simulink model "ConstrainedSphereModel"  (R2017b)
settings: Solver=VariableStepAuto  StartTime=0.0  StopTime=12  RelTol=1e-3
undefined symbols (not defined in the file): b_contact, C_F_alpha, C_F_kappa, g, k_contact, radiusRW, sigbuilder_block, theta_0, X, xPla, Y, yPla, Z
libraries: nesl_utility x15, sm_lib x7, vrlib x7, Parts_Lib x1, simulink x1
settings Model: Creator=r_ahmed_afzal  LastModifiedBy=r_ahmed_afzal

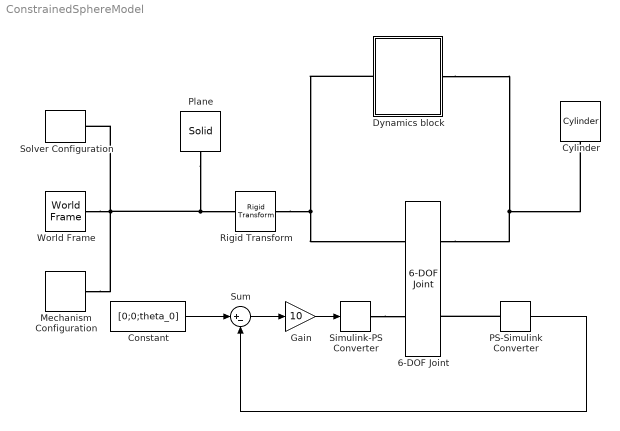
== system ConstrainedSphereModel ==
  6-DOF Joint : sm_lib/Joints/6-DOF Joint  SenseConstraintForce=off  SenseConstraintForceX=off  SenseConstraintForceY=off  SenseConstraintForceZ=off  SenseConstraintTorque=off  SenseConstraintTorqueX=off  SenseConstraintTorqueY=off  SenseConstraintTorqueZ=off  SenseTotalForce=off  SenseTotalForceX=off  SenseTotalForceY=off  SenseTotalForceZ=off  SenseTotalTorque=off  SenseTotalTorqueX=off  SenseTotalTorqueY=off  SenseTotalTorqueZ=off  CompositeWrenchDir=FollowerOnBase  CompositeWrenchFrame=BaseFrame  PxEquilibriumPosition=0  PxEquilibriumPositionUnits=m  PxSpringStiffness=0  PxSpringStiffnessUnits=N/m  PxDampingCoefficient=0  PxDampingCoefficientUnits=N/(m/s)  PxTorqueActuationMode=NoTorque  PxMotionActuationMode=ComputedMotion  PxSensePosition=off  PxSenseVelocity=off  PxSenseAcceleration=off  PxSenseTorqueForce=off  PxPositionTargetSpecify=on  PxPositionTargetPriority=High  PxPositionTargetValue=radiusRW  PxPositionTargetValueUnits=m  PxVelocityTargetSpecify=off  PxVelocityTargetPriority=High  PxVelocityTargetValue=0  PxVelocityTargetValueUnits=m/s  PyEquilibriumPosition=0  PyEquilibriumPositionUnits=m  PySpringStiffness=0  PySpringStiffnessUnits=N/m  PyDampingCoefficient=0  PyDampingCoefficientUnits=N/(m/s)  PyTorqueActuationMode=NoTorque  PyMotionActuationMode=ComputedMotion  PySensePosition=off  PySenseVelocity=off  PySenseAcceleration=off  PySenseTorqueForce=off  PyPositionTargetSpecify=on  PyPositionTargetPriority=High  PyPositionTargetValue=-xPla/2 + 0.1  PyPositionTargetValueUnits=m  PyVelocityTargetSpecify=off  PyVelocityTargetPriority=High  PyVelocityTargetValue=0  PyVelocityTargetValueUnits=m/s  PzEquilibriumPosition=0  PzEquilibriumPositionUnits=m  PzSpringStiffness=0  PzSpringStiffnessUnits=N/m  PzDampingCoefficient=0  PzDampingCoefficientUnits=N/(m/s)  PzTorqueActuationMode=NoTorque  PzMotionActuationMode=ComputedMotion  PzSensePosition=off  PzSenseVelocity=off  PzSenseAcceleration=off  PzSenseTorqueForce=off  PzPositionTargetSpecify=off  PzPositionTargetPriority=High  PzPositionTargetValue=0  PzPositionTargetValueUnits=m  PzVelocityTargetSpecify=off  PzVelocityTargetPriority=High  PzVelocityTargetValue=0  PzVelocityTargetValueUnits=m/s  SphDefPosRotationMethod=None  SphDefPosRotationAngleUnits=deg  SphDefPosRotationStandardAxis=+Z  SphDefPosRotationAngle=0.0  SphDefPosRotationArbitraryAxis=[0 0 1]  SphDefPosFollAlignAxisA=+X  SphDefPosBaseAlignAxisA=+Y  SphDefPosFollAlignAxisB=+Y  SphDefPosBaseAlignAxisB=+Z  SphDefPosRotationSequenceAxes=FollowerAxes  SphDefPosRotationSequence=XYX  SphDefPosRotationSequenceAngles=[0 0 0]  SphDefPosRotationSequenceAnglesUnits=deg  SphDefPosRotationMatrix=[1 0 0; 0 1 0; 0 0 1]  SphEqPosRotationMethod=None  SphEqPosRotationAngleUnits=deg  SphEqPosRotationStandardAxis=+Z  SphEqPosRotationAngle=0.0  SphEqPosRotationArbitraryAxis=[0 0 1]  SphEqPosFollAlignAxisA=+X  SphEqPosBaseAlignAxisA=+Y  SphEqPosFollAlignAxisB=+Y  SphEqPosBaseAlignAxisB=+Z  SphEqPosRotationSequenceAxes=FollowerAxes  SphEqPosRotationSequence=XYX  SphEqPosRotationSequenceAngles=[0 0 0]  SphEqPosRotationSequenceAnglesUnits=deg  SphEqPosRotationMatrix=[1 0 0; 0 1 0; 0 0 1]  SphSpringStiffness=0  SphSpringStiffnessUnits=N*m/deg  SphDampingCoefficient=0  SphDampingCoefficientUnits=N*m/(deg/s)  SphActuateTorqueX=off  SphActuateTorqueY=off  SphActuateTorqueZ=off  SphActuateTorque=on  SphTorqueActuationMode=InputTorque  SphMotionActuationMode=ComputedMotion  SphActuationFrame=FollowerFrame  SphSensePosition=off  SphSenseVelocityX=off  SphSenseVelocityY=off  SphSenseVelocityZ=off  SphSenseVelocity=on  SphSenseAccelerationX=off  SphSenseAccelerationY=off  SphSenseAccelerationZ=off  SphSenseAcceleration=off  SphSenseTorqueX=off  SphSenseTorqueY=off  SphSenseTorqueZ=off  SphSenseTorqueForce=off  SphSensingFrame=FollowerFrame  SphPositionTargetRotationMethod=StandardAxis  SphPositionTargetRotationAngleUnits=deg  SphPositionTargetRotationStandardAxis=+Y  SphPositionTargetRotationAngle=5  SphPositionTargetRotationArbitraryAxis=[0 0 1]  SphPositionTargetFollAlignAxisA=+X  SphPositionTargetBaseAlignAxisA=+Y  SphPositionTargetFollAlignAxisB=+Y  SphPositionTargetBaseAlignAxisB=+Z  SphPositionTargetRotationSequenceAxes=FollowerAxes  SphPositionTargetRotationSequence=XYX  SphPositionTargetRotationSequenceAngles=[0 0 0]  SphPositionTargetRotationSequenceAnglesUnits=deg  SphPositionTargetRotationMatrix=[1 0 0; 0 1 0; 0 0 1]  SphPositionTargetSpecify=on  SphPositionTargetPriority=High  SphVelocityTargetValue=[0 0 0]  SphVelocityTargetValueUnits=deg/s  SphVelocityTargetSpecify=off  SphVelocityTargetPriority=High  SphVelocityTargetInFollowerFrame=on
  Constant : Constant  Value=[0;0;theta_0]
  Cylinder : Parts_Lib/Cylinder  Tag=CustomStyle  cyl_radius=radiusRW  cyl_length=lengthRW  cyl_density=rhoRW  cyl_color=blue  cyl_opacity=1  cyl_color_custom="[0.7920    0.9900    0.9900]"  mark_radius=[0.75 0.5]  mark_len_factor=1.01  mark_angle=60  mark_color=purple  mark_opacity=1
  Dynamics block : Subsystem
  Gain : Gain  Gain=10
  Mechanism Configuration : sm_lib/Utilities/Mechanism Configuration  UniformGravity=Constant  GravityVector=[0 0 -g]  GravityUnits=m/s^2  LinearizationDelta=0.001
  PS-Simulink Converter : nesl_utility/PS-Simulink Converter  PhysicalDomain=network_engine_domain  SubClassName=ps_output  LeftPortType=input  RightPortType=output  PseudoPeriodic=off  Frequencies=[]  Unit=1  AffineConversion=off
  Plane : sm_lib/Body Elements/Solid  InertiaType=CalculateFromGeometry  Mass=1  MassUnits=kg  CenterOfMass=[0 0 0]  CenterOfMassUnits=m  MomentsOfInertia=[1 1 1]  MomentsOfInertiaUnits=kg*m^2  ProductsOfInertia=[1 1 1]  ProductsOfInertiaUnits=kg*m^2  DensityBased=on  Density=1000  DensityUnits=kg/m^3  DoExposeReferenceFrame=on  SerializedFrames=<Frames/>  GraphicType=FromGeometry  MarkerShape=Sphere  MarkerSize=10  GraphicVisPropType=SimpleVisualProperties  GraphicDiffuseColor=[0.5 0.5 0.5]  GraphicSpecularColor=[0.5 0.5 0.5 1.0]  GraphicAmbientColor=[0.15 0.15 0.15 1.0]  GraphicEmissiveColor=[0.0 0.0 0.0 1.0]  GraphicShininess=75  GraphicOpacity=0.5  GeometryShape=Brick  RectangleSize=[1 1]  RectangleSizeUnits=m  BrickDimensions=[xPla yPla 0.01]  BrickDimensionUnits=m  CylinderRadius=1  CylinderRadiusUnits=m  CylinderLength=1  CylinderLengthUnits=m  SphereRadius=1  SphereRadiusUnits=m  EllipsoidRadii=[1 1 1]  EllipsoidRadiiUnits=m  ExtrusionCrossSection=[1 1; -1 1; -1 -1; 1 -1]  ExtrusionCrossSectionUnits=m  ExtrusionLength=1  ExtrusionLengthUnits=m  PolygonNumSides=3  PolygonOuterRadius=1  PolygonOuterRadiusUnits=m  ExtGeomFileType=STEP  ExtGeomFileUnits=m  RevolutionCrossSection=[1 1; 1 -1; 2 -1; 2 1]  RevolutionCrossSectionUnits=m  RevolutionExtent=Full  RevolutionAngle=180  RevolutionAngleUnits=deg
  Rigid Transform : sm_lib/Frames and Transforms/Rigid Transform  TranslationMethod=None  TranslationStandardOffset=0  TranslationLengthUnit=m  TranslationStandardAxis=+Z  TranslationCartesianOffset=[0 0 0]  TranslationROffset=0  TranslationROffsetUnits=m  TranslationZOffset=0  TranslationZOffsetUnits=m  TranslationThetaOffset=0  TranslationThetaOffsetUnits=deg  RotationMethod=AlignedAxes  RotationAngleUnits=deg  RotationStandardAxis=+Z  RotationAngle=0.0  RotationArbitraryAxis=[0 0 1]  FollAlignAxisA=+Z  BaseAlignAxisA=+Y  FollAlignAxisB=+Y  BaseAlignAxisB=+X  RotationSequenceAxes=FollowerAxes  RotationSequence=XYX  RotationSequenceAngles=[0 0 0]  RotationSequenceAnglesUnits=deg  RotationMatrix=[1 0 0; 0 1 0; 0 0 1]
  Simulink-PS Converter : nesl_utility/Simulink-PS Converter  PhysicalDomain=network_engine_domain  SubClassName=ps_input  LeftPortType=input  RightPortType=output  PseudoPeriodic=off  Frequencies=[]  NoiseDistribution=none  NoiseParameters=[]  Unit=1  AffineConversion=off  FilteringAndDerivatives=filter  SimscapeFilterOrder=2  InputFilterTimeConstant=0.001  UdotUserProvided=0
  Solver Configuration : nesl_utility/Solver Configuration  PhysicalDomain=network_engine_domain  SubClassName=solver  LeftPortType=input  RightPortType=generic  Accelerate=off  Tones=[]  Harmonics=[]  SimulateNoise=off  Profile=off  UseLocalSampling=off  EnableSwitchedLinearOptims=on  FrequencyDomain=off  UseCCode=off  RelTol=0.001  AbsTol=1e-06  MinStep=1e-09  ToWorkspace=off  RevertToSquareIcSolve=off  NumHomotopyIterations=100  PhasorMode=off  PhasorModeNumHarmonics=1  DoDC=off  ResidualTolerance=1e-09  UseLocalSolver=off  LocalSolverChoice=NE_BACKWARD_EULER_ADVANCER  LocalSolverSampleTime=0.001  DoFixedCost=off  MaxNonlinIter=3  MaxModeIter=2  LinearAlgebra=Sparse  DelaysMemoryBudget=1024  AutomaticFiltering=on  FilteringTimeConstant=0.001
  Sum : Sum  Inputs=|+-
  World Frame : sm_lib/Frames and Transforms/World Frame
  wires:
  Constant/1 -> Sum/1
  PS-Simulink Converter/1 -> Sum/2
  Sum/1 -> Gain/1
  Gain/1 -> Simulink-PS Converter/1
  connections:
  Mechanism Configuration/RConn1 -- World Frame/RConn1 -- Rigid Transform/LConn1 -- Plane/RConn1 -- Solver Configuration/RConn1
  Simulink-PS Converter/RConn1 -- 6-DOF Joint/LConn2
  Rigid Transform/RConn1 -- Dynamics block/LConn1 -- 6-DOF Joint/LConn1
  Cylinder/LConn1 -- Dynamics block/RConn1 -- 6-DOF Joint/RConn1
  PS-Simulink Converter/LConn1 -- 6-DOF Joint/RConn2

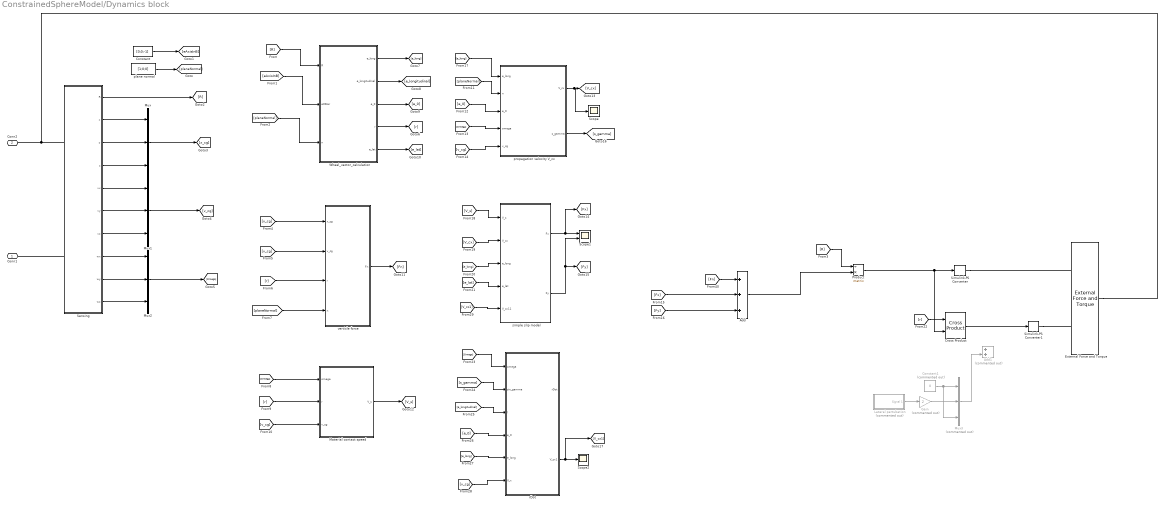
== system ConstrainedSphereModel/Dynamics block ==
  Add : Sum  Inputs=3
  Add1 : Sum  Commented=on
  Constant : Constant  Value=[0;0;-1]
  Constant1 : Constant  Commented=on  Value=0
  Cross Product : vrlib/Utilities/Cross Product
      settings: SourceProductBaseCode=VR
  External Force and Torque : sm_lib/Forces and Torques/External Force and Torque  ForceResolutionFrame=AttachedFrame  EnableForceX=off  EnableForceY=off  EnableForceZ=off  EnableForce=on  TorqueResolutionFrame=AttachedFrame  EnableTorqueX=off  EnableTorqueY=off  EnableTorqueZ=off  EnableTorque=on
  Gain : Gain  Commented=on  Gain=2
  Lateral pertubation : Subsystem  Tag=STV Subsys  Commented=on  LoadFcn=sigbuilder_block('load');  StartFcn=sigbuilder_block('start');  StopFcn=sigbuilder_block('stop');  ClipboardFcn=sigbuilder_block('clipboard');  mask(Sigbuilder block){tuvar=[0:10]}
      mask help: Simulink:masks:SigbuilderBlock_MD
      mask init:
      | if ~strcmp(get_param(bdroot(gcbh),'SimulationStatus'),'stopped') tuvar = sigbuilder_block('maskInit'); end
      settings: CopyFcn=sigbuilder_block('copy');  DeleteFcn=sigbuilder_block('delete');  ModelCloseFcn=sigbuilder_block('modelClose');  PreSaveFcn=sigbuilder_block('preSave');  PauseFcn=sigbuilder_block('pause');  ContinueFcn=sigbuilder_block('continue');  NameChangeFcn=sigbuilder_block('namechange');  OpenFcn=sigbuilder_block('open',[437.6 199.2 550.4 400 ]);  CloseFcn=sigbuilder_block('close');
      mask Display: plot(0, 0, 100, 100,[2, 2, 32, 32, 2], [68, 8, 8, 68, 68],[32, 2], [38, 38], [32, 19, 2],[53, 60, 44], [32, 17, 17, 2],[16, 16, 31, 31]);txt = getActiveGroup(gcbh);text(2, 100, txt,'verticalAlignment', 'top');
  Material contact speed : Subsystem
  Mux : Mux  Inputs=3
  Mux1 : Mux  Inputs=3
  Mux2 : Mux  Inputs=3
  Mux3 : Mux  Commented=on  Inputs=3
  Product : Product  Inputs=/*  Multiplication=Matrix(*)
  Scope : Scope
  Scope1 : Scope  NumInputPorts=2
  Scope2 : Scope
  Sensing : Subsystem
  Simulink-PS Converter : nesl_utility/Simulink-PS Converter  PhysicalDomain=network_engine_domain  SubClassName=ps_input  LeftPortType=input  RightPortType=output  PseudoPeriodic=off  Frequencies=[]  NoiseDistribution=none  NoiseParameters=[]  Unit=1  AffineConversion=off  FilteringAndDerivatives=provide  SimscapeFilterOrder=1  InputFilterTimeConstant=0.001  UdotUserProvided=0
  Simulink-PS Converter1 : nesl_utility/Simulink-PS Converter  PhysicalDomain=network_engine_domain  SubClassName=ps_input  LeftPortType=input  RightPortType=output  PseudoPeriodic=off  Frequencies=[]  NoiseDistribution=none  NoiseParameters=[]  Unit=1  AffineConversion=off  FilteringAndDerivatives=provide  SimscapeFilterOrder=1  InputFilterTimeConstant=0.001  UdotUserProvided=0
  Wheel_vector_calculation : Subsystem
  plane normal : Constant  Value=[1;0;0]
  propagation velocity V_cx : Subsystem
  rDot : Subsystem
  simple slip model : Subsystem
  verticle force : Subsystem
  Conn1 : PMIOPort  Port=1  Side=Left
  Conn2 : PMIOPort  Port=2  Side=Right
  wires:
  plane normal/1 -> [planeNormal]
  Constant/1 -> [eAxisInB]
  Sensing/1(R) -> [R]
  Sensing/2(x) -> Mux/1
  Sensing/3(y) -> Mux/2
  Sensing/4(z) -> Mux/3
  Mux/1 -> [x_cg]
  Sensing/6(vy) -> Mux1/2
  Sensing/5(vx) -> Mux1/1
  Sensing/7(vz) -> Mux1/3
  Mux1/1 -> [v_cg]
  Sensing/9(wy) -> Mux2/2
  Sensing/8(wx) -> Mux2/1
  Sensing/10(wz) -> Mux2/3
  Mux2/1 -> [Omega]
  [R] -> Product/1
  Product/1 -> Cross Product/2, Simulink-PS Converter/1
  [R] -> Wheel_vector_calculation/1(R)
  [eAxisInB] -> Wheel_vector_calculation/2(e0Star)
  [planeNormal] -> Wheel_vector_calculation/3(n)
  [x_cg] -> verticle force/1(x_cg)
  [v_cg] -> verticle force/2(v_cg)
  Wheel_vector_calculation/4(r) -> [r]
  Wheel_vector_calculation/1(e_long) -> [e_long]
  Wheel_vector_calculation/2(e_longitudinal) -> [e_longitudinal]
  Wheel_vector_calculation/3(e_0) -> [e_0]
  Wheel_vector_calculation/5(e_lat) -> [e_lat]
  [r] -> verticle force/3(r)
  [planeNormal] -> verticle force/4(n)
  verticle force/1(Fn) -> [Fn]
  [Omega] -> Material contact speed/1(omega)
  [r] -> Material contact speed/2(r)
  [v_cg] -> Material contact speed/3(v_cg)
  Material contact speed/1(V_s) -> [V_s]
  [Fn] -> Add/1
  [Fx] -> Add/2
  [Fy] -> Add/3
  [planeNormal] -> propagation velocity V_cx/2(n)
  [e_0] -> propagation velocity V_cx/3(e_0)
  [Omega] -> propagation velocity V_cx/4(omega)
  [v_cg] -> propagation velocity V_cx/5(v_cg)
  [e_long] -> propagation velocity V_cx/1(e_long)
  propagation velocity V_cx/1(V_cx) -> Scope/1, [V_cx]
  [V_s] -> simple slip model/1(V_s)
  [V_cx] -> simple slip model/2(V_cx)
  [e_long] -> simple slip model/3(e_long)
  [e_lat] -> simple slip model/4(e_lat)
  simple slip model/2(Fy) -> [Fy], Scope1/2
  Lateral pertubation/1(Signal 1) -> Gain/1
  Mux3/1 -> Add1/2
  Add/1 -> Product/2
  Gain/1 -> Mux3/2
  Constant1/1 -> Mux3/3, Mux3/1
  [r] -> Cross Product/1
  [Omega] -> rDot/1(omega)
  propagation velocity V_cx/2(s_gamma) -> [s_gamma]
  [s_gamma] -> rDot/2(sin_gamma)
  [e_longitudinal] -> rDot/3(l)
  [e_0] -> rDot/4(e_0)
  [e_long] -> rDot/5(e_long)
  [v_cg] -> rDot/6(V_x)
  rDot/2(V_cx1) -> [V_cx1], Scope2/1
  [V_cx1] -> simple slip model/5(V_cx11)
  simple slip model/1(Fx) -> [Fx], Scope1/1
  Cross Product/1 -> Simulink-PS Converter1/1
  connections:
  Sensing/LConn1 -- External Force and Torque/RConn1 -- Conn2/RConn1
  Sensing/LConn2 -- Conn1/RConn1
  Simulink-PS Converter/RConn1 -- External Force and Torque/LConn1
  Simulink-PS Converter1/RConn1 -- External Force and Torque/LConn2

== system ConstrainedSphereModel/Dynamics block/Lateral pertubation ==
  Demux : Demux  Tag=STV Demux  Outputs=1
  FromWs : FromWorkspace  Tag=STV FromWs  VariableName=tuvar  SampleTime=0
      SigBuilderData=|
      | common.afterFinalStr = 'Extrapolate'
      | common.sampleTime = 0
      | dataSet.timeRange = [0 10]
      | dataSet.name = 'Group 1'
      | sbobj.Groups.Name = 'Group 1'
      | sbobj.Groups.Signals.Name = 'Signal 1'
      | sbobj.Groups.Signals.XData = [0 1 1 1.5 1.5 10]
      | sbobj.Groups.Signals.YData = [0 0 1 1 0 0]
  Signal 1 : Outport  Tag=STV Outport
  wires:
  Demux/1 -> Signal 1/1
  FromWs/1 -> Demux/1

== system ConstrainedSphereModel/Dynamics block/Material contact speed ==
  omega : Inport
  r : Inport  Port=2
  v_cg : Inport  Port=3
  Cross Product : vrlib/Utilities/Cross Product
      settings: SourceProductBaseCode=VR
  Sum : Sum  Inputs=|++
  V_s : Outport
  wires:
  omega/1 -> Cross Product/1
  r/1 -> Cross Product/2
  Cross Product/1 -> Sum/1
  v_cg/1 -> Sum/2
  Sum/1 -> V_s/1

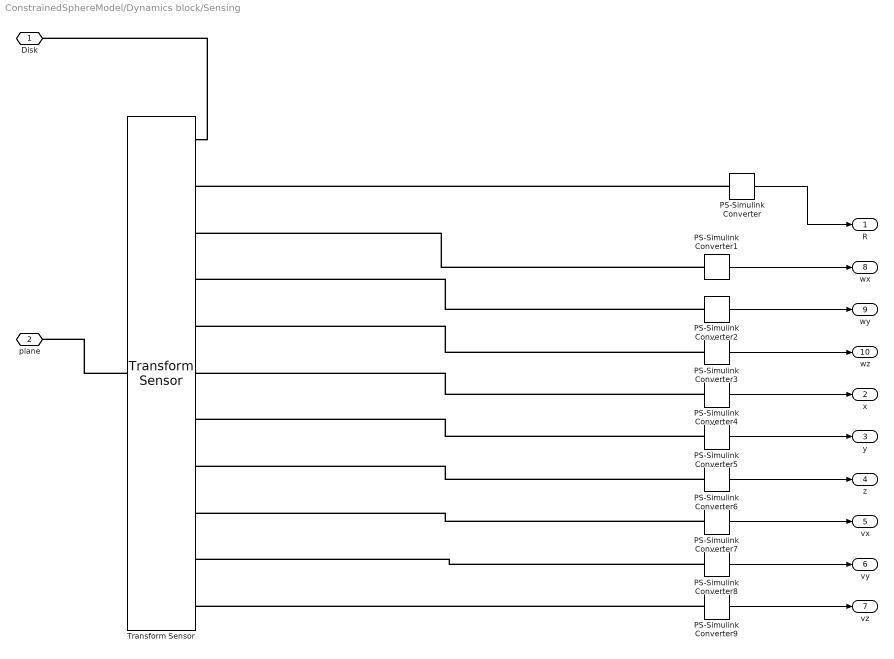
== system ConstrainedSphereModel/Dynamics block/Sensing ==
  PS-Simulink Converter{,1..9} (10 alike) : nesl_utility/PS-Simulink Converter  PhysicalDomain=network_engine_domain  SubClassName=ps_output  LeftPortType=input  RightPortType=output  PseudoPeriodic=off  Frequencies=[]  Unit=1  AffineConversion=off
  Transform Sensor : sm_lib/Frames and Transforms/Transform Sensor  MeasurementFrame=Base  SenseAngle=off  SenseAxis=off  SenseAngle1=off  SenseAngle2=off  SenseAngle3=off  SenseQ=off  SenseR=on  SenseOmegaX=on  SenseOmegaY=on  SenseOmegaZ=on  SenseOmega1=off  SenseOmega2=off  SenseOmega3=off  SenseQDot=off  SenseRDot=off  SenseAlphaX=off  SenseAlphaY=off  SenseAlphaZ=off  SenseAlpha1=off  SenseAlpha2=off  SenseAlpha3=off  SenseQDDot=off  SenseRDDot=off  SenseX=on  SenseY=on  SenseZ=on  SenseRad=off  SenseAzim=off  SenseDist=off  SenseInc=off  SenseXDot=on  SenseYDot=on  SenseZDot=on  SenseRadDot=off  SenseAzimDot=off  SenseDistDot=off  SenseIncDot=off  SenseXDDot=off  SenseYDDot=off  SenseZDDot=off  SenseRadDDot=off  SenseAzimDDot=off  SenseDistDDot=off  SenseIncDDot=off
  Disk : PMIOPort  Port=1  Side=Left
  plane : PMIOPort  Port=2  Side=Left
  R : Outport
  x : Outport  Port=2
  y : Outport  Port=3
  z : Outport  Port=4
  vx : Outport  Port=5
  vy : Outport  Port=6
  vz : Outport  Port=7
  wx : Outport  Port=8
  wy : Outport  Port=9
  wz : Outport  Port=10
  wires:
  PS-Simulink Converter/1 -> R/1
  PS-Simulink Converter4/1 -> x/1
  PS-Simulink Converter7/1 -> vx/1
  PS-Simulink Converter9/1 -> vz/1
  PS-Simulink Converter5/1 -> y/1
  PS-Simulink Converter6/1 -> z/1
  PS-Simulink Converter1/1 -> wx/1
  PS-Simulink Converter3/1 -> wz/1
  PS-Simulink Converter8/1 -> vy/1
  PS-Simulink Converter2/1 -> wy/1
  connections:
  PS-Simulink Converter8/LConn1 -- Transform Sensor/RConn10
  PS-Simulink Converter9/LConn1 -- Transform Sensor/RConn11
  PS-Simulink Converter7/LConn1 -- Transform Sensor/RConn9
  PS-Simulink Converter2/LConn1 -- Transform Sensor/RConn4
  PS-Simulink Converter1/LConn1 -- Transform Sensor/RConn3
  PS-Simulink Converter6/LConn1 -- Transform Sensor/RConn8
  PS-Simulink Converter4/LConn1 -- Transform Sensor/RConn6
  PS-Simulink Converter5/LConn1 -- Transform Sensor/RConn7
  Transform Sensor/RConn1 -- Disk/RConn1
  Transform Sensor/LConn1 -- plane/RConn1
  PS-Simulink Converter/LConn1 -- Transform Sensor/RConn2
  PS-Simulink Converter3/LConn1 -- Transform Sensor/RConn5

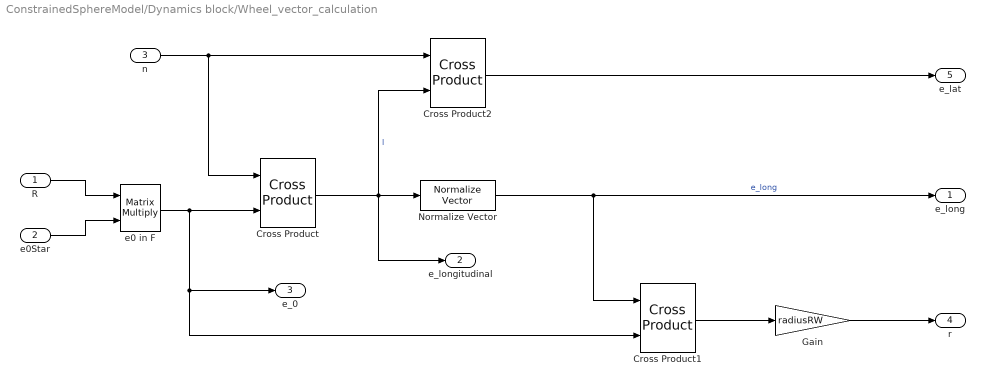
== system ConstrainedSphereModel/Dynamics block/Wheel_vector_calculation ==
  R : Inport
  e0Star : Inport  Port=2
  n : Inport  Port=3
  Cross Product : vrlib/Utilities/Cross Product
      settings: SourceProductBaseCode=VR
  Cross Product1 : vrlib/Utilities/Cross Product
      settings: SourceProductBaseCode=VR
  Cross Product2 : vrlib/Utilities/Cross Product
      settings: SourceProductBaseCode=VR
  Gain : Gain  Gain=radiusRW
  Normalize Vector : vrlib/Utilities/Normalize Vector  maxzero=0
      settings: SourceProductName=Simulink 3D Animation  SourceProductBaseCode=VR
  e0 in F : Product  Multiplication=Matrix(*)
  e_long : Outport
  e_longitudinal : Outport  Port=2
  e_0 : Outport  Port=3
  r : Outport  Port=4
  e_lat : Outport  Port=5
  wires:
  R/1 -> e0 in F/1
  e0Star/1 -> e0 in F/2
  e0 in F/1 -> e_0/1, Cross Product1/2, Cross Product/2
  n/1 -> Cross Product2/1, Cross Product/1
  Cross Product/1 -> Cross Product2/2, e_longitudinal/1, Normalize Vector/1  "l"
  Normalize Vector/1 -> Cross Product1/1, e_long/1  "e_long"
  Cross Product1/1 -> Gain/1
  Gain/1 -> r/1
  Cross Product2/1 -> e_lat/1

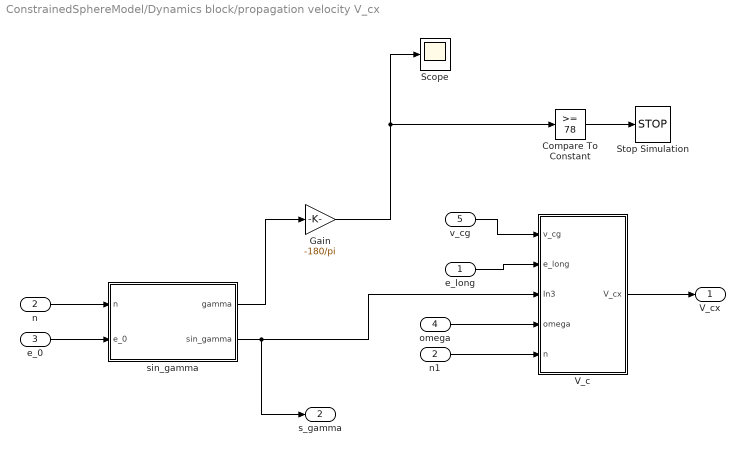
== system ConstrainedSphereModel/Dynamics block/propagation velocity V_cx ==
  e_long : Inport
  n : Inport  Port=2
  e_0 : Inport  Port=3
  omega : Inport  Port=4
  v_cg : Inport  Port=5
  Compare To Constant : simulink/Logic and Bit Operations/Compare To Constant  relop=>=  const=78  OutDataTypeStr=boolean
  Gain : Gain  Gain=-180/pi
  Scope : Scope
  Stop Simulation : Stop
  V_c : Subsystem
  n1 : InportShadow  Port=2
  sin_gamma : Subsystem
  V_cx : Outport
  s_gamma : Outport  Port=2
  wires:
  n/1 -> sin_gamma/1(n)
  e_0/1 -> sin_gamma/2(e_0)
  sin_gamma/1(gamma) -> Gain/1
  v_cg/1 -> V_c/1(v_cg)
  e_long/1 -> V_c/2(e_long)
  sin_gamma/2(sin_gamma) -> s_gamma/1, V_c/3(In3)
  omega/1 -> V_c/4(omega)
  n1/1 -> V_c/5(n)
  V_c/1(V_cx) -> V_cx/1
  Gain/1 -> Scope/1, Compare To Constant/1
  Compare To Constant/1 -> Stop Simulation/1

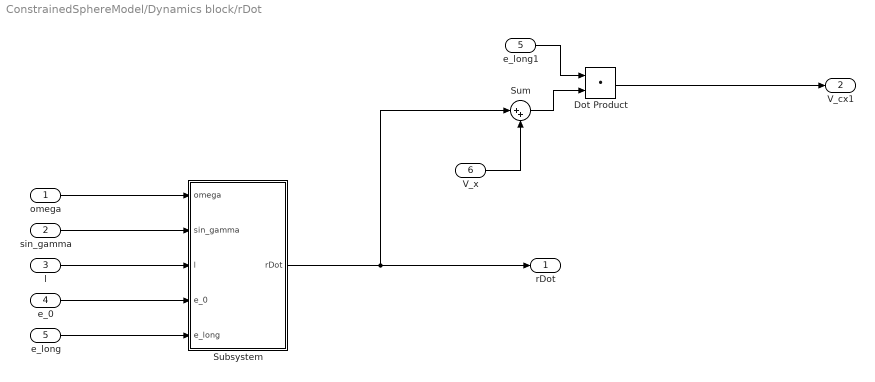
== system ConstrainedSphereModel/Dynamics block/rDot ==
  omega : Inport
  sin_gamma : Inport  Port=2
  l : Inport  Port=3
  e_0 : Inport  Port=4
  e_long : Inport  Port=5
  V_x : Inport  Port=6
  Dot Product : DotProduct  InputSameDT=on  OutDataTypeStr=Inherit: Inherit via internal rule
  Subsystem : Subsystem
  Sum : Sum  Inputs=|++
  e_long1 : InportShadow  Port=5
  rDot : Outport
  V_cx1 : Outport  Port=2
  wires:
  omega/1 -> Subsystem/1(omega)
  sin_gamma/1 -> Subsystem/2(sin_gamma)
  l/1 -> Subsystem/3(l)
  e_0/1 -> Subsystem/4(e_0)
  e_long/1 -> Subsystem/5(e_long)
  Subsystem/1(rDot) -> Sum/1, rDot/1
  V_x/1 -> Sum/2
  e_long1/1 -> Dot Product/1
  Sum/1 -> Dot Product/2
  Dot Product/1 -> V_cx1/1

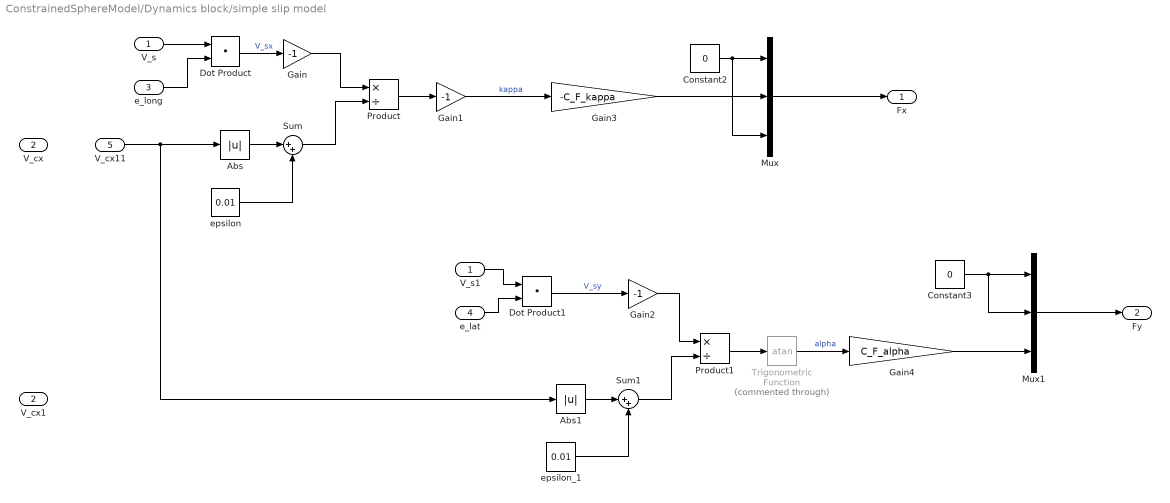
== system ConstrainedSphereModel/Dynamics block/simple slip model ==
  V_s : Inport
  V_cx : Inport  Port=2
  e_long : Inport  Port=3
  e_lat : Inport  Port=4
  V_cx11 : Inport  Port=5
  Abs : Abs
  Abs1 : Abs
  Constant2 : Constant  Value=0
  Constant3 : Constant  Value=0
  Dot Product : DotProduct  InputSameDT=on  OutDataTypeStr=Inherit: Inherit via internal rule
  Dot Product1 : DotProduct  InputSameDT=on  OutDataTypeStr=Inherit: Inherit via internal rule
  Gain : Gain  Gain=-1
  Gain1 : Gain  Gain=-1
  Gain2 : Gain  Gain=-1
  Gain3 : Gain  Gain=-C_F_kappa
  Gain4 : Gain  Gain=C_F_alpha
  Mux : Mux  Inputs=3
  Mux1 : Mux  Inputs=3
  Product : Product  Inputs=*/
  Product1 : Product  Inputs=*/
  Sum : Sum  Inputs=|++
  Sum1 : Sum  Inputs=|++
  Trigonometric Function : Trigonometry  Commented=through  Operator=atan
  V_cx1 : InportShadow  Port=2
  V_s1 : InportShadow
  epsilon : Constant  Value=0.01
  epsilon_1 : Constant  Value=0.01
  Fx : Outport
  Fy : Outport  Port=2
  wires:
  V_s/1 -> Dot Product/1
  e_long/1 -> Dot Product/2
  Dot Product/1 -> Gain/1  "V_sx"
  Gain/1 -> Product/1
  epsilon/1 -> Sum/2
  Sum/1 -> Product/2
  Product/1 -> Gain1/1
  Abs/1 -> Sum/1
  Gain1/1 -> Gain3/1  "kappa"
  V_s1/1 -> Dot Product1/1
  e_lat/1 -> Dot Product1/2
  Dot Product1/1 -> Gain2/1  "V_sy"
  Gain2/1 -> Product1/1
  epsilon_1/1 -> Sum1/2
  Sum1/1 -> Product1/2
  Abs1/1 -> Sum1/1
  Product1/1 -> Trigonometric Function/1
  Trigonometric Function/1 -> Gain4/1  "alpha"
  Mux/1 -> Fx/1
  Gain4/1 -> Mux1/3
  Gain3/1 -> Mux/2
  Constant2/1 -> Mux/3, Mux/1
  Constant3/1 -> Mux1/2, Mux1/1
  Mux1/1 -> Fy/1
  V_cx11/1 -> Abs1/1, Abs/1

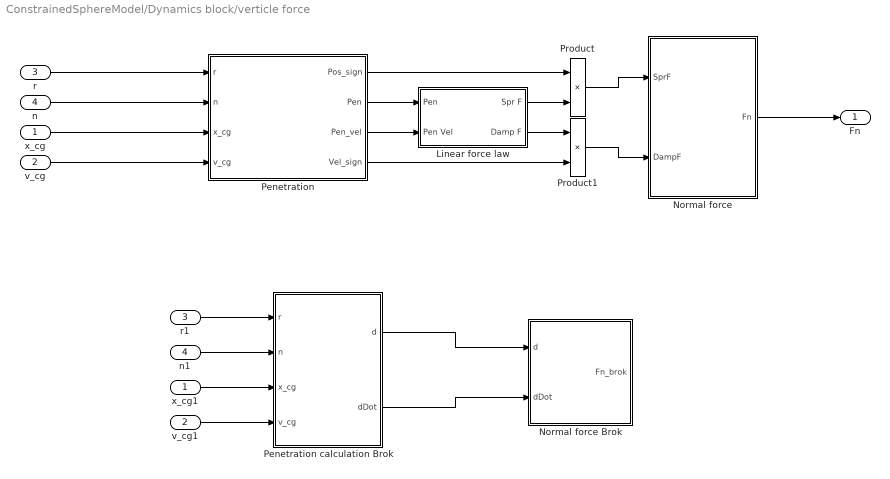
== system ConstrainedSphereModel/Dynamics block/verticle force ==
  x_cg : Inport
  v_cg : Inport  Port=2
  r : Inport  Port=3
  n : Inport  Port=4
  Linear force law : Subsystem  AncestorBlock=Contact_Forces_Lib/Force Law/Linear  VariantControl=Linear  mask(Linear Force Law){k_pen=k_contact, b_penvel=b_contact}
      mask prompts: k_pen "Contact Stiffness"; b_penvel "Contact Damping"
      mask help: Implements a contact force law as a linear spring damper. The damping force is applied only as the penetration depth increases.
      mask Help: web(which('Force_Laws.html'));
  Normal force : Subsystem
  Normal force Brok : Subsystem
  Penetration : Subsystem
  Penetration calculation Brok : Subsystem
  Product : Product
  Product1 : Product
  n1 : InportShadow  Port=4
  r1 : InportShadow  Port=3
  v_cg1 : InportShadow  Port=2
  x_cg1 : InportShadow
  Fn : Outport
  wires:
  x_cg/1 -> Penetration/3(x_cg)
  v_cg/1 -> Penetration/4(v_cg)
  Penetration/2(Pen) -> Linear force law/1(Pen)
  Penetration/3(Pen_vel) -> Linear force law/2(Pen Vel)
  Linear force law/1(Spr F) -> Product/2
  Penetration/1(Pos_sign) -> Product/1
  Linear force law/2(Damp F) -> Product1/1
  Penetration/4(Vel_sign) -> Product1/2
  Product/1 -> Normal force/1(SprF)
  Product1/1 -> Normal force/2(DampF)
  Normal force/1(Fn) -> Fn/1
  n/1 -> Penetration/2(n)
  r/1 -> Penetration/1(r)
  r1/1 -> Penetration calculation Brok/1(r)
  x_cg1/1 -> Penetration calculation Brok/3(x_cg)
  v_cg1/1 -> Penetration calculation Brok/4(v_cg)
  Penetration calculation Brok/1(d) -> Normal force Brok/1(d)
  Penetration calculation Brok/2(dDot) -> Normal force Brok/2(dDot)
  n1/1 -> Penetration calculation Brok/2(n)

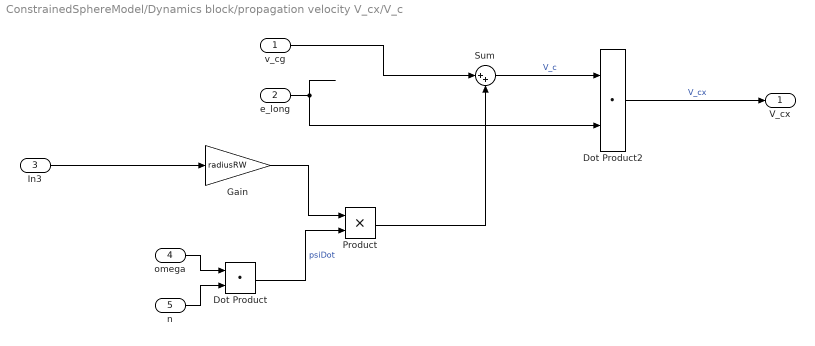
== system ConstrainedSphereModel/Dynamics block/propagation velocity V_cx/V_c ==
  v_cg : Inport
  e_long : Inport  Port=2
  In3 : Inport  Port=3
  omega : Inport  Port=4
  n : Inport  Port=5
  Dot Product : DotProduct  InputSameDT=on  OutDataTypeStr=Inherit: Inherit via internal rule
  Dot Product2 : DotProduct  InputSameDT=on  OutDataTypeStr=Inherit: Inherit via internal rule
  Gain : Gain  Gain=radiusRW
  Product : Product
  Sum : Sum  Inputs=|++
  V_cx : Outport
  wires:
  n/1 -> Dot Product/2
  Gain/1 -> Product/1
  Product/1 -> Sum/2
  Dot Product2/1 -> V_cx/1  "V_cx"
  Sum/1 -> Dot Product2/1  "V_c"
  Dot Product/1 -> Product/2  "psiDot"
  In3/1 -> Gain/1
  omega/1 -> Dot Product/1
  v_cg/1 -> Sum/1
  e_long/1 -> Dot Product2/2

== system ConstrainedSphereModel/Dynamics block/propagation velocity V_cx/sin_gamma ==
  n : Inport
  e_0 : Inport  Port=2
  Dot Product : DotProduct  InputSameDT=on  OutDataTypeStr=Inherit: Inherit via internal rule
  Gain : Gain  Gain=180/pi
  Scope : Scope
  Trigonometric Function : Trigonometry  Operator=asin
  gamma : Outport
  sin_gamma : Outport  Port=2
  wires:
  Gain/1 -> Scope/1
  n/1 -> Dot Product/1
  Trigonometric Function/1 -> gamma/1, Gain/1
  e_0/1 -> Dot Product/2
  Dot Product/1 -> sin_gamma/1, Trigonometric Function/1  "sin_gamma"

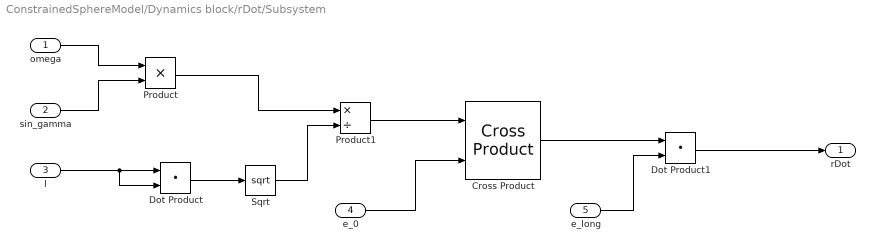
== system ConstrainedSphereModel/Dynamics block/rDot/Subsystem ==
  omega : Inport
  sin_gamma : Inport  Port=2
  l : Inport  Port=3
  e_0 : Inport  Port=4
  e_long : Inport  Port=5
  Cross Product : vrlib/Utilities/Cross Product
      settings: SourceProductBaseCode=VR
  Dot Product : DotProduct  InputSameDT=on  OutDataTypeStr=Inherit: Inherit via internal rule
  Dot Product1 : DotProduct  InputSameDT=on  OutDataTypeStr=Inherit: Inherit via internal rule
  Product : Product
  Product1 : Product  Inputs=*/
  Sqrt : Sqrt  SaturateOnIntegerOverflow=on
  rDot : Outport
  wires:
  sin_gamma/1 -> Product/2
  Cross Product/1 -> Dot Product1/1
  e_long/1 -> Dot Product1/2
  omega/1 -> Product/1
  Dot Product1/1 -> rDot/1
  Product/1 -> Product1/1
  Dot Product/1 -> Sqrt/1
  l/1 -> Dot Product/2, Dot Product/1
  Sqrt/1 -> Product1/2
  Product1/1 -> Cross Product/1
  e_0/1 -> Cross Product/2

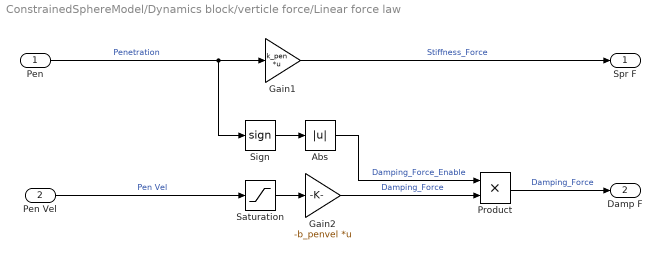
== system ConstrainedSphereModel/Dynamics block/verticle force/Linear force law ==
  Pen : Inport
  Pen Vel : Inport  Port=2
  Abs : Abs  ZeroCross=off
  Gain1 : Gain  Gain=k_pen  Multiplication=Matrix(K*u)  SaturateOnIntegerOverflow=on  OutDataTypeStr=Inherit: Same as input  ParamDataTypeStr=Inherit: Same as input
  Gain2 : Gain  Gain=-b_penvel  Multiplication=Matrix(K*u)  SaturateOnIntegerOverflow=on  OutDataTypeStr=Inherit: Same as input  ParamDataTypeStr=Inherit: Same as input
  Product : Product  RndMeth=Zero
  Saturation : Saturate  UpperLimit=Inf  LowerLimit=0  ZeroCross=off
  Sign : Signum  ZeroCross=off
  Spr F : Outport
  Damp F : Outport  Port=2
  wires:
  Saturation/1 -> Gain2/1
  Pen/1 -> Sign/1, Gain1/1  "Penetration"
  Abs/1 -> Product/1  "Damping_Force_Enable"
  Product/1 -> Damp F/1  "Damping_Force"
  Sign/1 -> Abs/1
  Pen Vel/1 -> Saturation/1  "Pen Vel"
  Gain2/1 -> Product/2  "Damping_Force"
  Gain1/1 -> Spr F/1  "Stiffness_Force"

== system ConstrainedSphereModel/Dynamics block/verticle force/Normal force ==
  SprF : Inport
  DampF : Inport  Port=2
  Add : Sum
  Constant : Constant  Value=0
  Mux : Mux  Inputs=3
  Fn : Outport
  wires:
  SprF/1 -> Add/1
  DampF/1 -> Add/2
  Add/1 -> Mux/1
  Constant/1 -> Mux/2, Mux/3
  Mux/1 -> Fn/1

== system ConstrainedSphereModel/Dynamics block/verticle force/Normal force Brok ==
  d : Inport
  dDot : Inport  Port=2
  Constant : Constant  Value=0
  Gain : Gain  Gain=k_contact
  Gain1 : Gain  Gain=b_contact
  Mux : Mux  Inputs=3
  Sum : Sum
  Fn_brok : Outport
  wires:
  d/1 -> Gain/1
  Gain/1 -> Sum/1
  dDot/1 -> Gain1/1
  Gain1/1 -> Sum/2
  Constant/1 -> Mux/2, Mux/3
  Sum/1 -> Mux/1
  Mux/1 -> Fn_brok/1

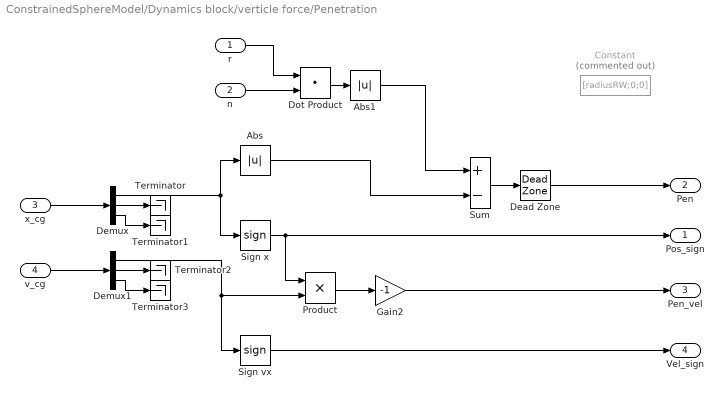
== system ConstrainedSphereModel/Dynamics block/verticle force/Penetration ==
  r : Inport
  n : Inport  Port=2
  x_cg : Inport  Port=3
  v_cg : Inport  Port=4
  Abs : Abs  ZeroCross=off
  Abs1 : Abs
  Constant : Constant  Commented=on  Value=[radiusRW;0;0]
  Dead Zone : DeadZone  LowerValue=-inf  UpperValue=0  SaturateOnIntegerOverflow=on
  Demux : Demux  Outputs=3
  Demux1 : Demux  Outputs=3
  Dot Product : DotProduct  InputSameDT=on  OutDataTypeStr=Inherit: Inherit via internal rule
  Gain2 : Gain  Gain=-1
  Product : Product
  Sign vx : Signum  ZeroCross=off
  Sign x : Signum  ZeroCross=off
  Sum : Sum  Inputs=+-
  Terminator{,1..3} (4 alike) : Terminator
  Pos_sign : Outport
  Pen : Outport  Port=2
  Pen_vel : Outport  Port=3
  Vel_sign : Outport  Port=4
  wires:
  Demux1/3 -> Terminator3/1
  Demux/2 -> Terminator/1
  Gain2/1 -> Pen_vel/1
  Dead Zone/1 -> Pen/1
  Sign x/1 -> Pos_sign/1, Product/1
  Demux1/1 -> Product/2, Sign vx/1
  Abs/1 -> Sum/2
  Product/1 -> Gain2/1
  Sign vx/1 -> Vel_sign/1
  Demux/1 -> Sign x/1, Abs/1
  Sum/1 -> Dead Zone/1
  Demux/3 -> Terminator1/1
  Demux1/2 -> Terminator2/1
  x_cg/1 -> Demux/1
  v_cg/1 -> Demux1/1
  n/1 -> Dot Product/2
  Dot Product/1 -> Abs1/1
  r/1 -> Dot Product/1
  Abs1/1 -> Sum/1

== system ConstrainedSphereModel/Dynamics block/verticle force/Penetration calculation Brok ==
  r : Inport
  n : Inport  Port=2
  x_cg : Inport  Port=3
  v_cg : Inport  Port=4
  Derivative : Derivative
  Dot Product : DotProduct  InputSameDT=on  OutDataTypeStr=Inherit: Inherit via internal rule
  Sum : Sum
  d : Outport
  dDot : Outport  Port=2
  wires:
  r/1 -> Sum/1
  x_cg/1 -> Sum/2
  Sum/1 -> Dot Product/1
  n/1 -> Dot Product/2
  Dot Product/1 -> d/1, Derivative/1  "d"
  Derivative/1 -> dDot/1
